simulink model "Motor"  (R2013a)
settings: Solver=FixedStepDiscrete  SolverMode=SingleTasking  StartTime=0.0  StopTime=inf  FixedStep=.03  RelTol=1e-3
undefined symbols (not defined in the file): sigbuilder_block
libraries: arduinolib x3
settings Model: SimulationMode=external  ExtModeTrigDuration=2  Creator=Alec  LastModifiedBy=user
settings OptimizationCC: ExpressionDepthLimit=2147483647  OptimizeModelRefInitCode=on  LifeSpan=1
settings DebuggingCC: SolverPrmCheckMsg=none  StrictBusMsg=Warning
settings HardwareCC: ProdBitPerInt=16  ProdBitPerPointer=8  ProdIntDivRoundTo=Zero  ProdEndianess=LittleEndian  ProdWordSize=8  ProdHWDeviceType=Atmel->AVR
settings RTWCC: SystemTargetFile=realtime.tlc  GenerateMakefile=off  TemplateMakefile=realtime.tmf  Description=Real-Time Toolbox  RTWVerbose=off  ProcessScript=realtime_make_rtw_hook
settings CodeAppCC: CustomSymbolStrType=$N$R$M  InternalIdentifier=Classic
settings STFCustomTargetCC: TargetLibSuffix=.a  GenerateSampleERTMain=on  ERTCustomFileBanners=on  SupportNonInlinedSFcns=off  SupportVariableSizeSignals=on  MATLABClassNameForMDSCustomization=Simulink.SoftwareTarget.ERTCustomization  SystemTargetFile=realtime.tlc
settings ERTTargetCC: ParMdlRefBuildCompliant=off  CompOptLevelCompliant=off  ConcurrentExecutionCompliant=off  CombineOutputUpdateFcns=off  ERTFirstTimeCompliant=off  SupportContinuousTime=on  SupportVariableSizeSignals=on  ModelStepFunctionPrototypeControlCompliant=off  CPPClassGenCompliant=off  ExtMode=on  ExtModeTransport=3  ExtModeMexFile=ext_serial_win32_comm  ExtModeMexArgs=0 12 115200  ERTSrcFileBannerTemplate=realtime_code_template.cgt  ERTHdrFileBannerTemplate=realtime_code_template.cgt  ERTDataSrcFileTemplate=realtime_code_template.cgt  ERTDataHdrFileTemplate=realtime_code_template.cgt  ERTCustomFileTemplate=realtime_file_process.tlc

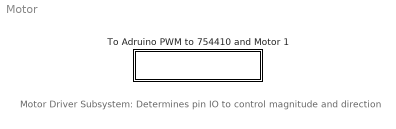
== system Motor ==
  note: Motor Driver Subsystem:
      | Determines pin IO to control
      | magnitude and direction
  To Adruino PWM to 754410 and Motor 1 : Subsystem

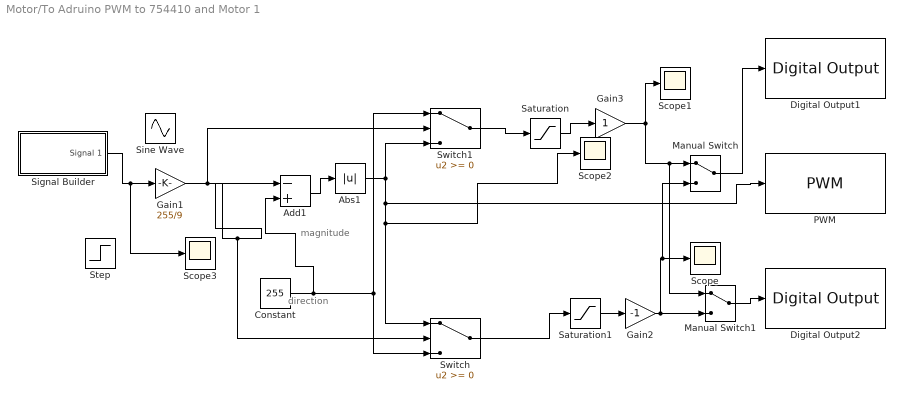
== system Motor/To Adruino PWM to 754410 and Motor 1 ==
  note: magnitude
  note: direction
  Abs1 : Abs
  Add1 : Sum  Inputs=-+
  Constant : Constant  Value=255
  Digital Output1 : arduinolib/Digital Output  pinNumber=6
  Digital Output2 : arduinolib/Digital Output  pinNumber=7
  Gain1 : Gain  Gain=255/9
  Gain2 : Gain  Gain=-1
  Gain3 : Gain
  Manual Switch : ManualSwitch
  Manual Switch1 : ManualSwitch
  PWM : arduinolib/PWM  pinNumber=5
  Saturation : Saturate  UpperLimit=255  LowerLimit=0
  Saturation1 : Saturate  UpperLimit=255  LowerLimit=0
  Scope{,1..3} (4 alike) : Scope
      Scope settings: TimeRange=10  YMin=226.667  YMax=226.667
      Scope1 settings: YMin=-300  YMax=300
      Scope2 settings: YMin=226.667  YMax=226.667  SaveName=ScopeData2
      Scope3 settings: YMin=1  YMax=1  SaveName=ScopeData3
  Signal Builder : Subsystem  Tag=STV Subsys  LoadFcn=sigbuilder_block('load');  StartFcn=sigbuilder_block('start');  StopFcn=sigbuilder_block('stop');  ClipboardFcn=sigbuilder_block('clipboard');  mask(Sigbuilder block){}
      mask help: Simulink:masks:SigbuilderBlock_MD
      mask init:
      | if ~strcmp(get_param(bdroot(gcbh),'SimulationStatus'),'stopped') tuvar = sigbuilder_block('maskInit'); end
      settings: CopyFcn=sigbuilder_block('copy');  DeleteFcn=sigbuilder_block('delete');  ModelCloseFcn=sigbuilder_block('modelClose');  PreSaveFcn=sigbuilder_block('preSave');  PauseFcn=sigbuilder_block('pause');  ContinueFcn=sigbuilder_block('continue');  NameChangeFcn=sigbuilder_block('namechange');  OpenFcn=sigbuilder_block('open',[437.25 118.5 550.5 372.75 ]);  CloseFcn=sigbuilder_block('close');
      mask Display: plot(0, 0, 100, 100,[2, 2, 32, 32, 2], [68, 8, 8, 68, 68],[32, 2], [38, 38], [32, 19, 2],[53, 60, 44], [32, 17, 17, 2],[16, 16, 31, 31]);txt = getActiveGroup(gcbh);text(2, 100, txt,'verticalAlignment', 'top');
  Sine Wave : Sin  Amplitude=7.4  Frequency=100  SampleTime=0
  Step : Step  Time=10  After=10  SampleTime=0
  Switch : Switch
  Switch1 : Switch
  wires:
  Gain1/1 -> Switch1/2, Add1/1, Switch/2
  Constant/1 -> Switch/3, Switch1/1, Add1/2
  Switch/1 -> Saturation1/1
  Switch1/1 -> Saturation/1
  Gain3/1 -> Manual Switch1/1, Manual Switch/1, Scope1/1
  Saturation1/1 -> Gain2/1
  Signal Builder/1(Signal 1) -> Scope3/1, Gain1/1
  Gain2/1 -> Manual Switch/2, Scope/1, Manual Switch1/2
  Abs1/1 -> PWM/1, Switch/1, Scope2/1, Switch1/3
  Saturation/1 -> Gain3/1
  Add1/1 -> Abs1/1
  Manual Switch/1 -> Digital Output1/1
  Manual Switch1/1 -> Digital Output2/1

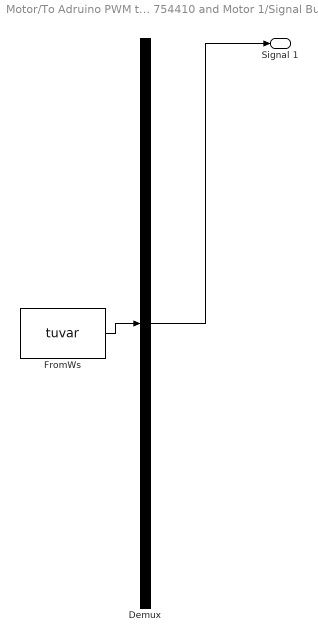
== system Motor/To Adruino PWM to 754410 and Motor 1/Signal Builder ==
  Demux : Demux  Tag=STV Demux  Outputs=1
  FromWs : FromWorkspace  Tag=STV FromWs  VariableName=tuvar  SampleTime=0
      SigBuilderData=|
      | common.afterFinalStr = 'Extrapolate'
      | common.sampleTime = 0
      | dataSet.timeRange = [0 10]
      | dataSet.name = 'Group 1'
      | sbobj.Groups.Name = 'Group 1'
      | sbobj.Groups.Signals.Name = 'Signal 1'
      | sbobj.Groups.Signals.XData = [0 1 1 5 5 6 10]
      | sbobj.Groups.Signals.YData = [1 1 -1 -1 1 1 1]
  Signal 1 : Outport  Tag=STV Outport
  wires:
  Demux/1 -> Signal 1/1
  FromWs/1 -> Demux/1
